simulink model "Conduction"  (R2016b)
settings: Solver=VariableStepAuto  StartTime=0.0  StopTime=0.08  RelTol=1e-3
libraries: powerlib x32, powerlib_meascontrol x5
settings Model: Creator=Youssef  LastModifiedBy=Youssef

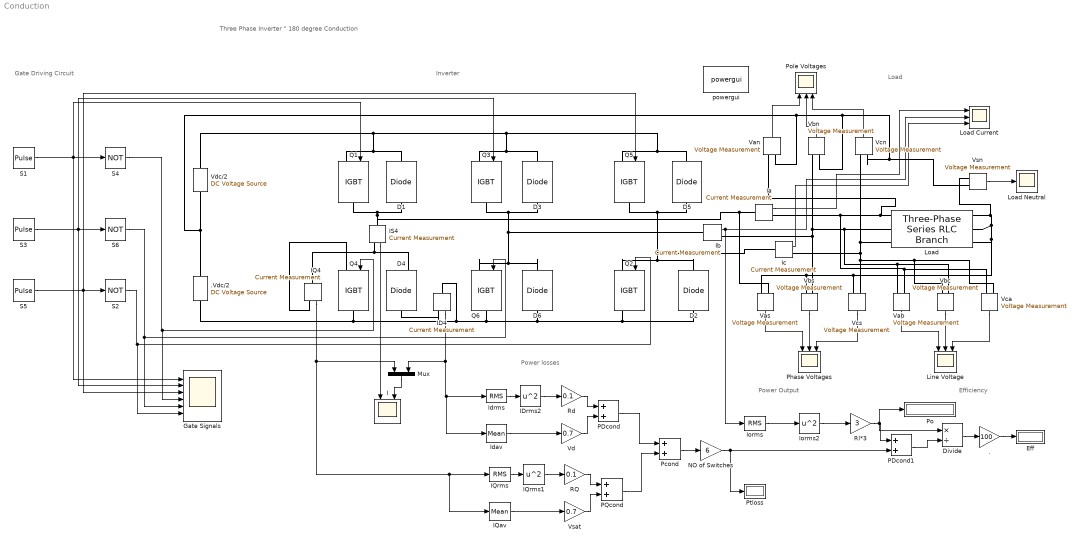
== system Conduction ==
  note: Gate Driving Circuit
  note: Load
  note: Three Phase Inverter " 180 degree Conduction
  note: Inverter
  note: Power losses
  note: Power Output
  note: Efficiency
  . : Gain  Gain=100
  .Vdc/2 : powerlib/Electrical Sources/DC Voltage Source  Amplitude=141  Measurements=None
  D{1..3,5..6} (5 alike) : powerlib/Power Electronics/Diode  Ron=0.001  Lon=0  Vf=0.8  IC=0  UseSnubber=off  Rs=500  Cs=250e-9  Measurements=off
  D4 : powerlib/Power Electronics/Diode  Ron=0.001  Lon=0  Vf=0.8  IC=0  UseSnubber=off  Rs=500  Cs=250e-9  Measurements=on
  Divide : Product  Inputs=*/  SaturateOnIntegerOverflow=on  RndMeth=Zero
  Eff : Display
  Gate Signals : Scope  NumInputPorts=6
  I : Scope  NumInputPorts=2
  ID4 : powerlib/Measurements/Current Measurement  PhasorSimulation=off  OutputType=Complex  PSBequivalent=0
  IDrms2 : Math  Operator=square  SaturateOnIntegerOverflow=on
  IQ4 : powerlib/Measurements/Current Measurement  PhasorSimulation=off  OutputType=Complex  PSBequivalent=0
  IQav : powerlib_meascontrol/Measurements/Mean  Freq=50  Vinit=0  Ts=0
  IQrms : powerlib_meascontrol/Measurements/RMS  TrueRMS=on  Freq=50  RMSInit=0  Ts=0
  IQrms1 : Math  Operator=square  SaturateOnIntegerOverflow=on
  IS4 : powerlib/Measurements/Current Measurement  PhasorSimulation=off  OutputType=Complex  PSBequivalent=0
  Ia : powerlib/Measurements/Current Measurement  PhasorSimulation=off  OutputType=Complex  PSBequivalent=0
  Ib : powerlib/Measurements/Current Measurement  PhasorSimulation=off  OutputType=Complex  PSBequivalent=0
  Ic : powerlib/Measurements/Current Measurement  PhasorSimulation=off  OutputType=Complex  PSBequivalent=0
  Idav : powerlib_meascontrol/Measurements/Mean  Freq=50  Vinit=0  Ts=0
  Idrms : powerlib_meascontrol/Measurements/RMS  TrueRMS=on  Freq=50  RMSInit=0  Ts=0
  Iorms : powerlib_meascontrol/Measurements/RMS  TrueRMS=on  Freq=50  RMSInit=0  Ts=0
  Iorms2 : Math  Operator=square  SaturateOnIntegerOverflow=on
  Line Voltage : Scope  NumInputPorts=3
  Load : powerlib/Elements/Three-Phase Series RLC Branch  LConnTagsString=A|B|C  RConnTagsString=A|B|C  BranchType=RL  Resistance=1  Inductance=1e-3  Capacitance=1e-6  Measurements=None
  Load Current : Scope  NumInputPorts=3
  Load Neutral : Scope
  Mux : Mux  Inputs=2
  NO of Switches : Gain  Gain=6
  PDcond : Sum
  PDcond1 : Sum
  PQcond : Sum
  Pcond : Sum
  Phase Voltages : Scope  NumInputPorts=3
  Po : Display
  Pole Voltages : Scope  NumInputPorts=3
  "Ptloss " : Display
  Q{1,3..6} (5 alike) : powerlib/Power Electronics/IGBT  Ron=0.001  Lon=0  Vf=0.4  Tf=1e-6  Tt=2e-6  IC=0  Rs=1e5  Cs=inf  Measurements=off
  Q2 : powerlib/Power Electronics/IGBT  Ron=0.001  Lon=0  Vf=0.4  Tf=1e-6  Tt=2e-6  IC=0  Rs=1e5  Cs=inf  Measurements=on
  RQ : Gain  Gain=0.1
  Rd : Gain  Gain=0.1
  Rl*3 : Gain  Gain=3
  S1 : DiscretePulseGenerator  PulseType=Time based  Period=0.02  PulseWidth=50
  S2 : Logic  Operator=NOT  AllPortsSameDT=off  OutDataTypeStr=boolean
  S3 : DiscretePulseGenerator  PulseType=Time based  Period=0.02  PulseWidth=50  PhaseDelay=0.02/3
  S4 : Logic  Operator=NOT  AllPortsSameDT=off  OutDataTypeStr=boolean
  S5 : DiscretePulseGenerator  PulseType=Time based  Period=0.02  PulseWidth=50  PhaseDelay=(2*0.02)/3
  S6 : Logic  Operator=NOT  AllPortsSameDT=off  OutDataTypeStr=boolean
  Vab : powerlib/Measurements/Voltage Measurement  PhasorSimulation=off  OutputType=Complex  PSBequivalent=0
  Van : powerlib/Measurements/Voltage Measurement  PhasorSimulation=off  OutputType=Complex  PSBequivalent=0
  Vas : powerlib/Measurements/Voltage Measurement  PhasorSimulation=off  OutputType=Complex  PSBequivalent=0
  Vbc : powerlib/Measurements/Voltage Measurement  PhasorSimulation=off  OutputType=Complex  PSBequivalent=0
  Vbn : powerlib/Measurements/Voltage Measurement  PhasorSimulation=off  OutputType=Complex  PSBequivalent=0
  Vbs : powerlib/Measurements/Voltage Measurement  PhasorSimulation=off  OutputType=Complex  PSBequivalent=0
  Vca : powerlib/Measurements/Voltage Measurement  PhasorSimulation=off  OutputType=Complex  PSBequivalent=0
  Vcn : powerlib/Measurements/Voltage Measurement  PhasorSimulation=off  OutputType=Complex  PSBequivalent=0
  Vcs : powerlib/Measurements/Voltage Measurement  PhasorSimulation=off  OutputType=Complex  PSBequivalent=0
  Vd : Gain  Gain=0.7
  Vdc/2 : powerlib/Electrical Sources/DC Voltage Source  Amplitude=141  Measurements=None
  Vsat : Gain  Gain=0.7
  Vsn : powerlib/Measurements/Voltage Measurement  PhasorSimulation=off  OutputType=Complex  PSBequivalent=0
  powergui : powerlib/powergui  Priority=1  SimulationMode=Discrete  SolverType=Tustin/Backward Euler (TBE)  SampleTime=1e-6  frequency=60  SPID=off  DisableSnubberDevices=off  DisableRonSwitches=off  DisableVfSwitches=off  SwTol=0  DisplayEquations=off  Interpol=off  ExternalGateDelay=off  methode=off  Ts=10  FunctionMessages=off  echomessages=off  HookPort=off  EnableUseOfTLC=off  x0status=blocks  frequencyindice=0  Pbase=100e6  ErrMax=1e-4  Iterations=50  UnitsV=kV  UnitsW=MW  buscounter=0  RestoreLinks=warning  ResistiveCurrentMeasurement=off  Frange=[0:2:500]  Ylog=off  Xlog=on  ShowGrid=off  save=off  variable=ZData  structure=I  ZoomFFT=off  StartTime=0.02  cycles=2  DisplayStyle=1  fundamental=50  FreqAxis=off  MaxFrequency=1000  frequencyindicesteady=1  RmsSteady=1  display=off
  wires:
  S1/1 -> Gate Signals/1, Q1/1, S4/1
  S3/1 -> Gate Signals/2, Q3/1, S6/1
  S5/1 -> Gate Signals/3, Q5/1, S2/1
  S6/1 -> Gate Signals/5, Q6/1
  Ia/1 -> Load Current/1
  Ib/1 -> Iorms/1, Load Current/2
  Ic/1 -> Load Current/3
  Van/1 -> Pole Voltages/1
  Vbn/1 -> Pole Voltages/2
  Vcn/1 -> Pole Voltages/3
  Vas/1 -> Phase Voltages/1
  Vbs/1 -> Phase Voltages/2
  Vcs/1 -> Phase Voltages/3
  Vab/1 -> Line Voltage/1
  Vbc/1 -> Line Voltage/2
  Vca/1 -> Line Voltage/3
  Vsn/1 -> Load Neutral/1
  S4/1 -> Gate Signals/4, Q4/1
  S2/1 -> Gate Signals/6, Q2/1
  ID4/1 -> Idav/1, Idrms/1, Mux/2
  Mux/1 -> I/2
  IS4/1 -> I/1
  Idrms/1 -> IDrms2/1
  IDrms2/1 -> Rd/1
  Idav/1 -> Vd/1
  Vd/1 -> PDcond/2
  Rd/1 -> PDcond/1
  IQ4/1 -> IQav/1, IQrms/1, Mux/1
  IQrms/1 -> IQrms1/1
  IQrms1/1 -> RQ/1
  IQav/1 -> Vsat/1
  Vsat/1 -> PQcond/2
  RQ/1 -> PQcond/1
  PQcond/1 -> Pcond/2
  PDcond/1 -> Pcond/1
  Pcond/1 -> NO of Switches/1
  Iorms/1 -> Iorms2/1
  Iorms2/1 -> Rl*3/1
  NO of Switches/1 -> "Ptloss "/1, PDcond1/2
  Rl*3/1 -> Divide/1, Po/1, PDcond1/1
  PDcond1/1 -> Divide/2
  Divide/1 -> ./1
  ./1 -> Eff/1
  connections:
  D1/RConn1 -- D5/RConn1 -- Q5/LConn1 -- Q3/LConn1 -- D3/RConn1 -- Vdc/2/RConn1 -- Q1/LConn1
  D4/RConn1 -- IS4/RConn1 -- IQ4/LConn1
  Q3/RConn1 -- Ib/LConn1 -- D6/RConn1 -- Q6/LConn1 -- D3/LConn1
  D5/LConn1 -- D2/RConn1 -- Q2/LConn1 -- Ic/LConn1 -- Q5/RConn1
  Vdc/2/LConn1 -- Vsn/LConn2 -- Vcn/LConn2 -- Vbn/LConn2 -- Van/LConn2 -- .Vdc/2/RConn1
  .Vdc/2/LConn1 -- ID4/LConn1 -- D2/LConn1 -- Q2/RConn1 -- D6/LConn1 -- Q6/RConn1 -- Q4/RConn1
  Load/RConn1 -- Vsn/LConn1 -- Vas/LConn2 -- Vbs/LConn2 -- Vcs/LConn2 -- Load/RConn3 -- Load/RConn2
  Ia/RConn1 -- Vca/LConn2 -- Vab/LConn1 -- Van/LConn1 -- Load/LConn1
  Ib/RConn1 -- Vab/LConn2 -- Vbc/LConn1 -- Load/LConn2 -- Vbn/LConn1 -- Vbs/LConn1
  Ic/RConn1 -- Vca/LConn1 -- Vbc/LConn2 -- Vcs/LConn1 -- Vcn/LConn1 -- Load/LConn3
  ID4/RConn1 -- D4/LConn1
  IQ4/RConn1 -- Q4/LConn1
  Q1/RConn1 -- Vas/LConn1 -- Ia/LConn1 -- IS4/LConn1 -- D1/LConn1
